simulink model "pe_dc_motor_control"  (R2018b)
settings: Solver=FixedStepDiscrete  StartTime=0.0  StopTime=4  FixedStep=Ts  MaxStep=1e-2  RelTol=1e-3  AbsTol=1e-3
PreLoadFcn:
  | pe_dc_motor_control_data;
undefined symbols (not defined in the file): fsw, ia_max, ia_min, Kb, Ki_i, Ki_n, Kp_i, Kp_n, Ra, Ts, Tsc
libraries: fl_lib x16, nesl_utility x8, pe_lib x2, peDcCurrentController x1, peDiscretePi x1, pePwmGenerator x1
Description:
  | DC Motor Control
  | 
  | This example shows a cascade speed-control structure for a DC motor.
  | A PWM controlled four-quadrant Chopper is used to feed the DC motor.
  | The Control subsystem includes the outer speed-control loop, the inner
  | current-control loop, and the PWM generation. The total simulation
  | time (t) is 4 seconds. At t = 1.5 seconds, the load torque increases.
  | At t = 2.5 seconds, the reference speed is changed from 1000 rpm to
  | 2000 rpm.
  | 
  | Copyright 2016-2017 The MathWorks, Inc.
settings Model: Creator=The MathWorks, Inc.  LastModifiedBy=Marko
settings SolverCC: AutoScaleAbsTol=off
settings OptimizationCC: LifeSpan=inf
settings DebuggingCC: UnderspecifiedInitializationDetection=Classic  MergeDetectMultiDrivingBlocksExec=none  LibraryContextMissingDiagnostic=none  SFUnexpectedBacktrackingDiag=warning  SFNoUnconditionalDefaultTransitionDiag=warning  SFExecutionAtInitializationDiag=none
settings SFSimCC: SimUseLocalCustomCode=off
settings RTWCC: RTWUseLocalCustomCode=off
settings CodeAppCC: StateflowObjectComments=on
settings GRTTargetCC: TargetLangStandard=C89/C90 (ANSI)  GeneratePreprocessorConditionals=Disable all
settings ConfigComp: CovMetricSettings=dw  CovHtmlReporting=on  CovSaveCumulativeToWorkspaceVar=on  CovSaveSingleToWorkspaceVar=on  CovExternalEMLEnable=off
settings SimscapeCC: SimscapeLogType=all  SimscapeLogSimulationStatistics=on  SimscapeLogName=simlog_pe_dc_motor_control  SimscapeLogLimitData=off

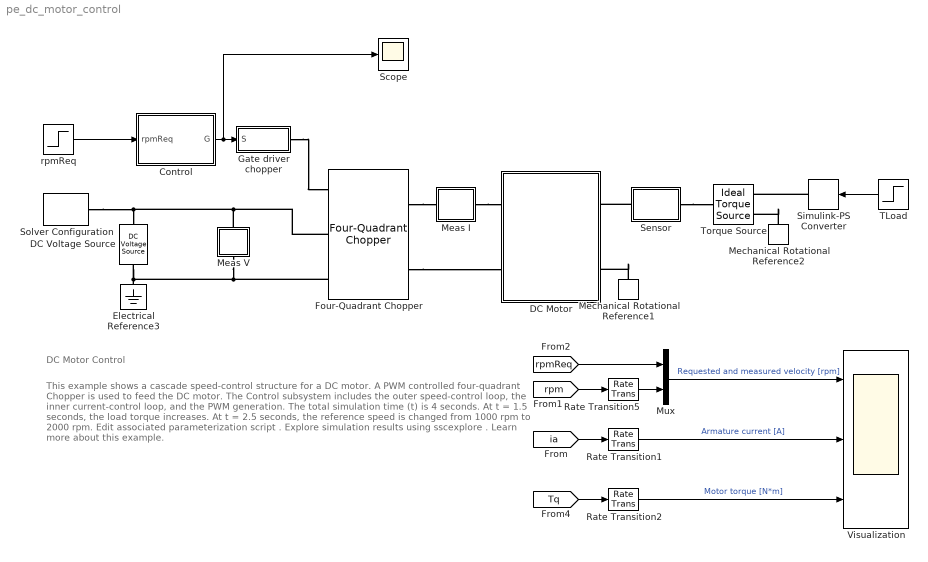
== system pe_dc_motor_control ==
  note: DC Motor Control
  note: This example shows a cascade speed-control structure for a DC motor. A PWM
      | controlled four-quadrant Chopper is used to feed the DC motor. The Control
      | subsystem includes the outer speed-control loop, the inner current-control loop, and
      | the PWM generation. The total simulation time (t) is 4 seconds. At t = 1.5 seconds,
      | the load torque increases. At t = 2.5 seconds, the reference speed is changed from
      | 1000 rpm to 2000 rpm.
      | Edit associated parameterization script .
      | Explore simulation results using sscexplore .
      | Learn more about this example.
  Control : Subsystem
  DC Motor : Subsystem
  DC Voltage Source : fl_lib/Electrical/Electrical Sources/DC Voltage Source  v0=15 V
      settings: SourceProductName=Foundation Library
  Electrical Reference3 : fl_lib/Electrical/Electrical Elements/Electrical Reference
      settings: SourceProductName=Foundation Library
  Four-Quadrant Chopper : pe_lib/Semiconductors/Four-Quadrant Chopper  device_type=3  Vf=0.8 V  Ron=0.001 Ohm  Rds=0.001 Ohm  Goff=1e-5 1/Ohm  Vth=0.5 V  Vgt=1 V  Vgt_off=-1 V  Ih=1 A  diode_param=2  diode_Vf=0.8 V  diode_Ron=0.001 Ohm  diode_Goff=1e-5 1/Ohm  diode_C=50 nF  diode_iRM=-235 A  diode_iF=300 A  diode_idot=-50 A/us  diode_trr_param=1  diode_trr_factor=3  diode_trr=15 us  diode_Qrr=1500 s*uA  snubber_type=0  Rs=0.1 Ohm  Cs=1e-7 F
      settings: SourceProductName=Simscape Power Systems  SourceProductBaseCode=PS
  Gate driver chopper : Subsystem
  Meas I : Subsystem
  Meas V : Subsystem
  Mechanical Rotational Reference1 : fl_lib/Mechanical/Rotational Elements/Mechanical Rotational Reference
      settings: SourceProductName=Foundation Library
  Mechanical Rotational Reference2 : fl_lib/Mechanical/Rotational Elements/Mechanical Rotational Reference
      settings: SourceProductName=Foundation Library
  Mux : Mux  Inputs=2
  Rate Transition1 : RateTransition
  Rate Transition2 : RateTransition  OutPortSampleTime=Tsc
  Rate Transition5 : RateTransition
  Scope : Scope
  Sensor : Subsystem
  Simulink-PS Converter : nesl_utility/Simulink-PS Converter  PhysicalDomain=network_engine_domain  SubClassName=ps_input  LeftPortType=input  RightPortType=output  PseudoPeriodic=off  Frequencies=[]  NoiseDistribution=none  NoiseParameters=[]  Unit=1  AffineConversion=off  FilteringAndDerivatives=provide  SimscapeFilterOrder=1  InputFilterTimeConstant=0.001  UdotUserProvided=0
  Solver Configuration : nesl_utility/Solver Configuration  PhysicalDomain=network_engine_domain  SubClassName=solver  LeftPortType=input  RightPortType=generic  Tones=[]  Harmonics=[]  SimulateNoise=off  Profile=off  UseLocalSampling=off  EnableSwitchedLinearOptims=on  FrequencyDomain=off  UseCCode=off  RelTol=0.001  AbsTol=1e-06  MinStep=1e-09  ToWorkspace=off  RevertToSquareIcSolve=off  NumHomotopyIterations=100  PhasorMode=off  PhasorModeNumHarmonics=1  DoDC=off  ResidualTolerance=1e-09  UseLocalSolver=on  LocalSolverChoice=NE_BACKWARD_EULER_ADVANCER  LocalSolverSampleTime=Ts  DoFixedCost=on  MaxNonlinIter=3  MaxModeIter=2  LinearAlgebra=auto  EquationFormulation=NE_TIME_EF  DelaysMemoryBudget=1024  AutomaticFiltering=on  FilteringTimeConstant=0.001  PartitionStorageMethod=AS_NEEDED  PartitionMemoryBudget=1024
  TLoad : Step  Time=1.5  After=-0.015  SampleTime=0
  Torque Source : fl_lib/Mechanical/Mechanical Sources/Ideal Torque Source
      settings: SourceProductName=Foundation Library
  Visualization : Scope  NumInputPorts=3
  rpmReq : Step  Time=2.5  Before=1000  After=2000  SampleTime=0
  wires:
  TLoad/1 -> Simulink-PS Converter/1
  rpmReq/1 -> Control/1(rpmReq)
  [rpm] -> Rate Transition5/1
  [rpmReq] -> Mux/1
  [ia] -> Rate Transition1/1
  Rate Transition5/1 -> Mux/2
  [Tq] -> Rate Transition2/1
  Mux/1 -> Visualization/1  "Requested and measured velocity [rpm]"
  Rate Transition1/1 -> Visualization/2  "Armature current [A]"
  Rate Transition2/1 -> Visualization/3  "Motor torque [N*m]"
  Control/1(G) -> Scope/1, Gate driver chopper/1(S)
  connections:
  Solver Configuration/RConn1 -- Four-Quadrant Chopper/LConn2 -- Meas V/LConn1 -- DC Voltage Source/LConn1
  Simulink-PS Converter/RConn1 -- Torque Source/RConn1
  Mechanical Rotational Reference2/LConn1 -- Torque Source/RConn2
  Electrical Reference3/LConn1 -- Meas V/RConn1 -- Four-Quadrant Chopper/LConn3 -- DC Voltage Source/RConn1
  Mechanical Rotational Reference1/LConn1 -- DC Motor/RConn2
  Four-Quadrant Chopper/RConn2 -- DC Motor/LConn2
  Four-Quadrant Chopper/RConn1 -- Meas I/LConn1
  Sensor/LConn1 -- DC Motor/RConn1
  Sensor/RConn1 -- Torque Source/LConn1
  Meas I/RConn1 -- DC Motor/LConn1
  Gate driver chopper/RConn1 -- Four-Quadrant Chopper/LConn1

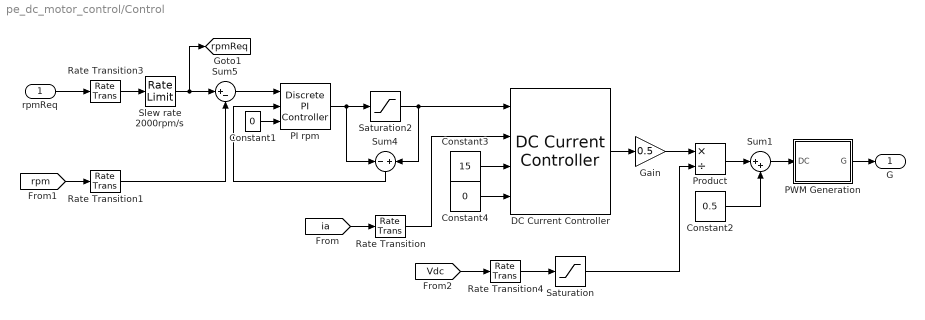
== system pe_dc_motor_control/Control ==
  rpmReq : Inport
  Constant1 : Constant  Value=0  SampleTime=Tsc
  Constant2 : Constant  Value=0.5  SampleTime=Tsc
  Constant3 : Constant  Value=15  SampleTime=Tsc
  Constant4 : Constant  Value=0  SampleTime=Tsc
  DC Current Controller : peDcCurrentController/DC Current Controller  Kp=Kp_i  Ki=Ki_i  Kaw=Kaw_i  VoltLim=Positive and negative voltage  Ts=Tsc  Tsd=0.001  ActZC=off
  Gain : Gain  Gain=0.5
  PI rpm : peDiscretePi/Discrete PI Controller  Kp=Kp_n  Ki=Ki_n  Kaw=Kaw_n  x0=0  Ts=Tsc
  PWM Generation : Subsystem
  Product : Product  Inputs=*/
  Rate Transition{,1,3..4} (4 alike) : RateTransition  OutPortSampleTime=Tsc
  Saturation : Saturate  UpperLimit=20  LowerLimit=0.5
  Saturation2 : Saturate  UpperLimit=ia_max  LowerLimit=ia_min
  Slew rate 2000rpm/s : RateLimiter  RisingSlewLimit=2000  FallingSlewLimit=-2000  SampleTimeMode=inherited
  Sum1 : Sum  Inputs=|++
  Sum4 : Sum  Inputs=-+
  Sum5 : Sum  Inputs=|+-
  G : Outport
  tag scope: rpmReq=global
  wires:
  PI rpm/1 -> Sum4/1, Saturation2/1
  Constant1/1 -> PI rpm/3
  Sum5/1 -> PI rpm/1
  Saturation/1 -> Product/2
  Sum4/1 -> PI rpm/2
  Saturation2/1 -> DC Current Controller/1, Sum4/2
  rpmReq/1 -> Rate Transition3/1
  Gain/1 -> Product/1
  Product/1 -> Sum1/1
  [rpm] -> Rate Transition1/1
  Slew rate 2000rpm/s/1 -> Sum5/1, [rpmReq]
  [Vdc] -> Rate Transition4/1
  Constant2/1 -> Sum1/2
  Rate Transition3/1 -> Slew rate 2000rpm/s/1
  [ia] -> Rate Transition/1
  Rate Transition4/1 -> Saturation/1
  Rate Transition1/1 -> Sum5/2
  Sum1/1 -> PWM Generation/1(DC)
  PWM Generation/1(G) -> G/1
  DC Current Controller/1 -> Gain/1
  Rate Transition/1 -> DC Current Controller/2
  Constant3/1 -> DC Current Controller/3
  Constant4/1 -> DC Current Controller/4

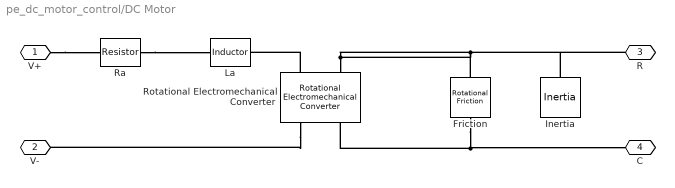
== system pe_dc_motor_control/DC Motor ==
  Friction : fl_lib/Mechanical/Rotational Elements/Rotational Friction  brkwy_trq=0.02e-3 N*m  brkwy_vel=0.1 rad/s  Col_trq=0.02e-3 N*m  visc_coef=Bm N*m/(rad/s)  w_specify=off  w_priority=None  w=0 rad/s  w_nominal_specify=off  w_nominal_unit=rad/s  w_nominal_value=1  t_specify=off  t_priority=None  t=0 N*m  t_nominal_specify=off  t_nominal_unit=N*m  t_nominal_value=1
      settings: SourceProductName=Foundation Library
  Inertia : fl_lib/Mechanical/Rotational Elements/Inertia  inertia=Jm kg*m^2  w_specify=off  w_priority=High  w=0 rad/s  w_nominal_specify=off  w_nominal_unit=rad/s  w_nominal_value=1  t_specify=off  t_priority=None  t=0 N*m  t_nominal_specify=off  t_nominal_unit=N*m  t_nominal_value=1
      settings: SourceProductName=Foundation Library
  La : fl_lib/Electrical/Electrical Elements/Inductor  l=La H  r=0 Ohm  g=1e-9 1/Ohm  i_specify=off  i_priority=None  i=0 A  i_nominal_specify=off  i_nominal_unit=A  i_nominal_value=1  v_specify=off  v_priority=None  v=0 V  v_nominal_specify=off  v_nominal_unit=V  v_nominal_value=1  i_L_specify=on  i_L_priority=High  i_L=0 A  i_L_nominal_specify=off  i_L_nominal_unit=A  i_L_nominal_value=1
      settings: SourceProductName=Foundation Library
  Ra : fl_lib/Electrical/Electrical Elements/Resistor  R=Ra Ohm  i_specify=off  i_priority=None  i=0 A  i_nominal_specify=off  i_nominal_unit=A  i_nominal_value=1  v_specify=off  v_priority=None  v=0 V  v_nominal_specify=off  v_nominal_unit=V  v_nominal_value=1
      settings: SourceProductName=Foundation Library
  Rotational Electromechanical Converter : fl_lib/Electrical/Electrical Elements/Rotational Electromechanical Converter  K=Kb V/(rad/s)  i_specify=off  i_priority=None  i=0 A  i_nominal_specify=off  i_nominal_unit=A  i_nominal_value=1  v_specify=off  v_priority=None  v=0 V  v_nominal_specify=off  v_nominal_unit=V  v_nominal_value=1  t_specify=off  t_priority=None  t=0 N*m  t_nominal_specify=off  t_nominal_unit=N*m  t_nominal_value=1  w_specify=off  w_priority=None  w=0 rad/s  w_nominal_specify=off  w_nominal_unit=rad/s  w_nominal_value=1
      settings: SourceProductName=Foundation Library
  V+ : PMIOPort  Side=Left
  V- : PMIOPort  Port=2  Side=Left
  R : PMIOPort  Port=3  Side=Right
  C : PMIOPort  Port=4  Side=Right
  connections:
  Ra/RConn1 -- La/LConn1
  Rotational Electromechanical Converter/RConn1 -- V-/RConn1
  Rotational Electromechanical Converter/LConn2 -- R/RConn1 -- Inertia/LConn1 -- Friction/LConn1
  V+/RConn1 -- Ra/LConn1
  Friction/RConn1 -- Rotational Electromechanical Converter/RConn2 -- C/RConn1
  Rotational Electromechanical Converter/LConn1 -- La/RConn1

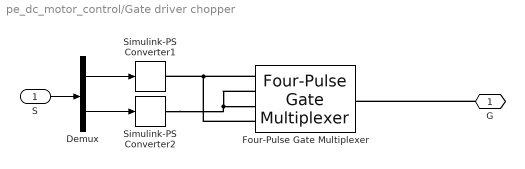
== system pe_dc_motor_control/Gate driver chopper ==
  S : Inport
  Demux : Demux  Outputs=2
  Four-Pulse Gate Multiplexer : pe_lib/Semiconductors/Four-Pulse Gate Multiplexer  R=0 Ohm
      settings: SourceProductName=Simscape Power Systems  SourceProductBaseCode=PS
  Simulink-PS Converter1 : nesl_utility/Simulink-PS Converter  PhysicalDomain=network_engine_domain  SubClassName=ps_input  LeftPortType=input  RightPortType=output  PseudoPeriodic=off  Frequencies=[]  NoiseDistribution=none  NoiseParameters=[]  Unit=1  AffineConversion=off  FilteringAndDerivatives=zero  SimscapeFilterOrder=1  InputFilterTimeConstant=0.001  UdotUserProvided=1
  Simulink-PS Converter2 : nesl_utility/Simulink-PS Converter  PhysicalDomain=network_engine_domain  SubClassName=ps_input  LeftPortType=input  RightPortType=output  PseudoPeriodic=off  Frequencies=[]  NoiseDistribution=none  NoiseParameters=[]  Unit=1  AffineConversion=off  FilteringAndDerivatives=zero  SimscapeFilterOrder=1  InputFilterTimeConstant=0.001  UdotUserProvided=1
  G : PMIOPort  Side=Right
  wires:
  Demux/2 -> Simulink-PS Converter2/1
  S/1 -> Demux/1
  Demux/1 -> Simulink-PS Converter1/1
  connections:
  Simulink-PS Converter2/RConn1 -- Four-Pulse Gate Multiplexer/LConn2 -- Four-Pulse Gate Multiplexer/LConn3
  Four-Pulse Gate Multiplexer/LConn1 -- Four-Pulse Gate Multiplexer/LConn4 -- Simulink-PS Converter1/RConn1
  G/RConn1 -- Four-Pulse Gate Multiplexer/RConn1

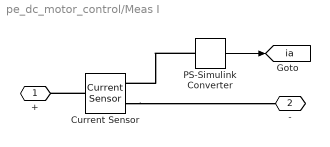
== system pe_dc_motor_control/Meas I ==
  Current Sensor : fl_lib/Electrical/Electrical Sensors/Current Sensor
      settings: SourceProductName=Foundation Library
  PS-Simulink Converter : nesl_utility/PS-Simulink Converter  PhysicalDomain=network_engine_domain  SubClassName=ps_output  LeftPortType=input  RightPortType=output  PseudoPeriodic=off  Frequencies=[]  Unit=1  AffineConversion=off
  + : PMIOPort  Side=Left
  - : PMIOPort  Port=2  Side=Right
  tag scope: ia=global
  wires:
  PS-Simulink Converter/1 -> [ia]
  connections:
  PS-Simulink Converter/LConn1 -- Current Sensor/RConn1
  Current Sensor/RConn2 -- -/RConn1
  Current Sensor/LConn1 -- +/RConn1

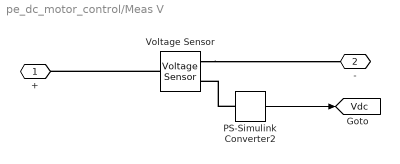
== system pe_dc_motor_control/Meas V ==
  PS-Simulink Converter2 : nesl_utility/PS-Simulink Converter  PhysicalDomain=network_engine_domain  SubClassName=ps_output  LeftPortType=input  RightPortType=output  PseudoPeriodic=off  Frequencies=[]  Unit=V  AffineConversion=off
  Voltage Sensor : fl_lib/Electrical/Electrical Sensors/Voltage Sensor
      settings: SourceProductName=Foundation Library
  + : PMIOPort  Side=Left
  - : PMIOPort  Port=2  Side=Right
  tag scope: Vdc=global
  wires:
  PS-Simulink Converter2/1 -> [Vdc]
  connections:
  Voltage Sensor/LConn1 -- +/RConn1
  PS-Simulink Converter2/LConn1 -- Voltage Sensor/RConn1
  Voltage Sensor/RConn2 -- -/RConn1

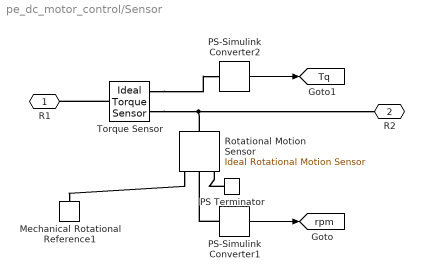
== system pe_dc_motor_control/Sensor ==
  Mechanical Rotational Reference1 : fl_lib/Mechanical/Rotational Elements/Mechanical Rotational Reference
      settings: SourceProductName=Foundation Library
  PS Terminator : fl_lib/Physical Signals/Sinks/PS Terminator
      settings: SourceProductName=Foundation Library
  PS-Simulink Converter1 : nesl_utility/PS-Simulink Converter  PhysicalDomain=network_engine_domain  SubClassName=ps_output  LeftPortType=input  RightPortType=output  PseudoPeriodic=off  Frequencies=[]  Unit=rpm  AffineConversion=off
  PS-Simulink Converter2 : nesl_utility/PS-Simulink Converter  PhysicalDomain=network_engine_domain  SubClassName=ps_output  LeftPortType=input  RightPortType=output  PseudoPeriodic=off  Frequencies=[]  Unit=N*m  AffineConversion=off
  Rotational Motion Sensor : fl_lib/Mechanical/Mechanical Sensors/Ideal Rotational Motion Sensor  offset=0 rad
      settings: SourceProductName=Foundation Library
  Torque Sensor : fl_lib/Mechanical/Mechanical Sensors/Ideal Torque Sensor
      settings: SourceProductName=Foundation Library
  R1 : PMIOPort  Side=Left
  R2 : PMIOPort  Port=2  Side=Right
  tag scope: Tq=global, rpm=global
  wires:
  PS-Simulink Converter2/1 -> [Tq]
  PS-Simulink Converter1/1 -> [rpm]
  connections:
  Rotational Motion Sensor/RConn1 -- Mechanical Rotational Reference1/LConn1
  Torque Sensor/LConn1 -- R1/RConn1
  Torque Sensor/RConn2 -- PS-Simulink Converter2/LConn1
  Rotational Motion Sensor/LConn1 -- R2/RConn1 -- Torque Sensor/RConn1
  PS-Simulink Converter1/LConn1 -- Rotational Motion Sensor/RConn2
  PS Terminator/LConn1 -- Rotational Motion Sensor/RConn3

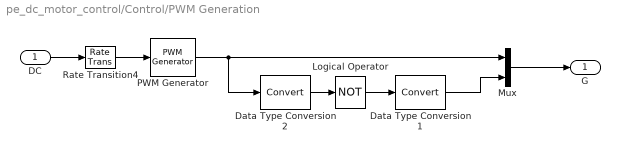
== system pe_dc_motor_control/Control/PWM Generation ==
  DC : Inport
  Data Type Conversion1 : DataTypeConversion
  Data Type Conversion2 : DataTypeConversion
  Logical Operator : Logic  Operator=NOT  AllPortsSameDT=off  OutDataTypeStr=boolean
  Mux : Mux  Inputs=2
  PWM Generator : pePwmGenerator/PWM Generator  CarrCount=Up  Tper=1/fsw  Ts=Ts
  Rate Transition4 : RateTransition  OutPortSampleTime=Ts
  G : Outport
  wires:
  Data Type Conversion2/1 -> Logical Operator/1
  DC/1 -> Rate Transition4/1
  PWM Generator/1 -> Mux/1, Data Type Conversion2/1
  Logical Operator/1 -> Data Type Conversion1/1
  Data Type Conversion1/1 -> Mux/2
  Mux/1 -> G/1
  Rate Transition4/1 -> PWM Generator/1
